simulink model "boost_converter1"  (R2022b)
settings: Solver=ode15s  StartTime=0.0  StopTime=2  RelTol=1e-3
libraries: spsSeriesRLCBranchLib x6, spsMosfetLib x5, spsCurrentMeasurementLib x4, spsVoltageMeasurementLib x4, spsPVArrayLib x1, spsDiodeLib x1, spspowerguiLib x1
settings Model: Creator=nisha  LastModifiedBy=nisha

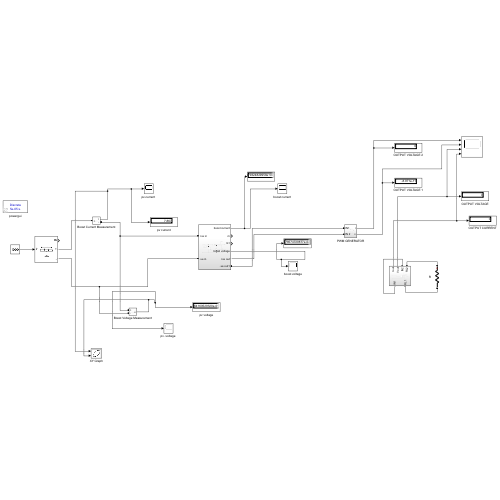
[thumbnail: Simulink's stored preview of the top-level diagram]
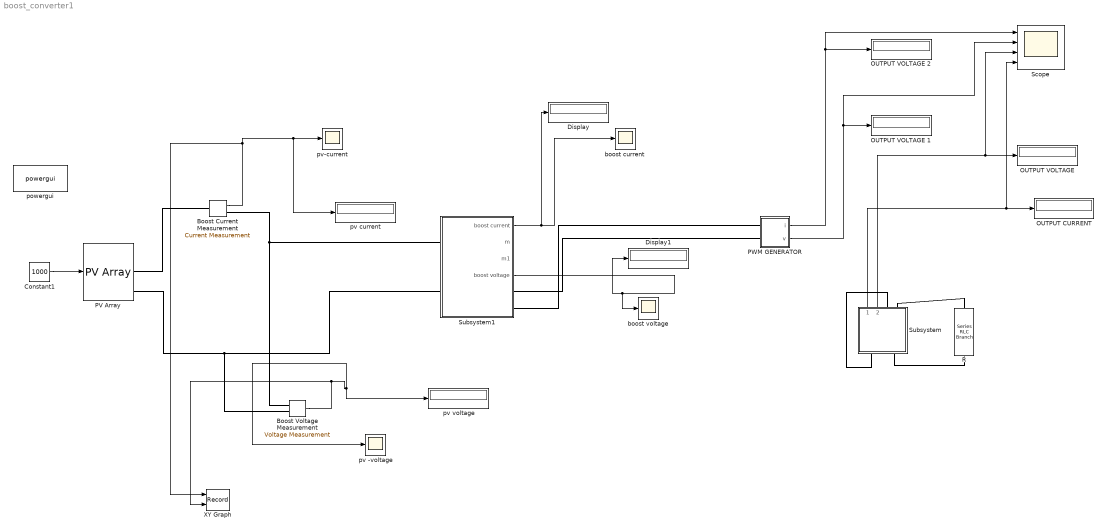
== system boost_converter1 ==
  Boost Current Measurement : spsCurrentMeasurementLib/Current Measurement  PhasorSimulation=off  OutputType=Complex  PSBequivalent=0
  Boost Voltage Measurement : spsVoltageMeasurementLib/Voltage Measurement  PhasorSimulation=off  OutputType=Complex  PSBequivalent=0
  Constant1 : Constant  Value=1000
  Display : Display
      settings: Format=long_e
  Display1 : Display
      settings: Format=long_e
  OUTPUT CURRENT : Display
  OUTPUT VOLTAGE : Display
  OUTPUT VOLTAGE 1 : Display
  OUTPUT VOLTAGE 2 : Display
  PV Array : spsPVArrayLib/PV Array  Npar=1  Nser=1  PlotType=array @ 1000 W/m2 & specified temperatures  S_vec="[ 1000  500  100 ]"  Temp_C_vec="[ 45 25  ]"  ModuleName=User-defined  PlotWhenSelected=off  Pm=213.15  Ncell=60  Voc=35  Isc=7.84  Vm=29  Im=7.35  beta_Voc_pc=-0.36099  alpha_Isc_pc=0.102  beta_Voc=-0.12635  alpha_Isc=0.0079968  IL=7.8812  I0=2.9282e-10  nI=0.94636  Rsh=184.8932  Rs=0.22133  RobustModel=on  RobustCellTemperature=25  BAL=on  Tc=1e-6  Tfilter=5e-5
  PWM GENERATOR : Subsystem
  R : spsSeriesRLCBranchLib/Series RLC Branch  LConnTagsString=__new0  RConnTagsString=__new0  BranchType=R  Resistance=1e-3  Inductance=10e-3  SetiL0=off  InitialCurrent=0  Capacitance=1e-6  Setx0=off  InitialVoltage=0  Measurements=None
  Scope : Scope  NumInputPorts=4
  Subsystem : Subsystem
  Subsystem1 : Subsystem
  XY Graph : Record  FileSettingsInternal="{\"entries\":[{\"content\":{\"excelSettings\":{\"content\":{},\"type\":\"Streamout.ExcelSettings\"}},\"type\":\"Streamout.FileSettingStorage\",\"uuid\":\"bb79825a-9a84-48d6-b614-86dd706c150b\"}],\"packageUris\":[\"http://schema.mathworks.com/mf0/streamout_blocks/R2020a\"],\"version\":\"1.0\"}"  Layout=[1 1]  SignalsInternal="{\"entries\":[{\"content\":{\"signals\":[{\"content\":{\"blockPath\":[\"boost_converter1/XY Graph\"],\"channel\":[],\"dimensions\":[1],\"domain\":\"boost_converter1/XY Graph\",\"lineColor\":\"#a2142f\",\"plots\":[1],\"port\":1,\"sid\":[],\"signalID\":8,\"signalName\":\"Boost Current Measurement\"},\"type\":\"RecordBlkView.Signal\",\"uuid\":\"aac8f88a-0a32-46b7-9f55-3afda7bd7b5f\"},{\"content\":{\"blockPath\":[\"boost_converter1/XY Graph\"],\"channel\":[],\"dimensions\":[1],\"domain\":\"boost_converter1/XY Graph\",\"lineColor\":\"#139fff\",\"plots\":[1],\"port\":2,\"sid\":[],\"signalID\":11,\"signalName\":\"Boost Voltage Measurement\"},\"type\":\"RecordBlkView.Signal\",\"uuid\":\"9a516fd9-1f24-4ca3-8a78-6277114d30cd\"}]},\"type\":\"RecordBlkView.InputSignals\",\"uuid\":\"dc6686e9-87f2-4b25-8e6b-96e90d879104\"}],\"packageUris\":[\"http://schema.mathworks.com/mf0/streamout_blocks/R2020a\"],\"version\":\"1.0\"}"  VisualizationBindings="{\"xyplotplugin\":{\"info\":[{\"series\":[{\"bindingParametersList\":[{\"parameter\":\"X-Axis\",\"signalID\":8,\"signalName\":\"Boost Current Measurement\"},{\"parameter\":\"Y-Axis\",\"signalID\":11,\"signalName\":\"Boost Voltage Measurement\"}],\"seriesID\":18183}],\"subplotID\":1}]}}"  CompatibilityTag=XY
  boost current : Scope
  boost voltage : Scope
  powergui : spspowerguiLib/powergui  Priority=1  SimulationMode=Discrete  SampleTime=5e-5  frequency=60  Iterations=50  frequencyindice=0  Pbase=100e6  ErrMax=1e-4  UnitsV=kV  UnitsW=MW  buscounter=0  FunctionMessages=off  echomessages=off  EnableUseOfTLC=off  CurrentSourceSwitches=off  DisableSnubberDevices=off  DisableRonSwitches=off  DisableVfSwitches=off  DisplayEquations=off  AutomaticDiscreteSolvers=off  SolverType=Tustin/Backward Euler (TBE)  Interpol=off  ExternalGateDelay=off  methode=off  Ts=100  x0status=blocks  SPID=on  SwTol=0  HookPort=off  NonlinearTolerance=1e-4  nMaxIteration=100  ContinueOnMaxIteration=off  RestoreLinks=warning  ResistiveCurrentMeasurement=off  Frange=[0:2:500]  Ylog=off  Xlog=on  ShowGrid=off  save=off  variable=ZData  structure=0  ZoomFFT=off  StartTime=0.0  cycles=1  DisplayStyle=1  fundamental=60  FreqAxis=off  MaxFrequency=1000  frequencyindicesteady=1  RmsSteady=1  display=off
  "pv -voltage " : Scope
  pv current : Display
  pv voltage : Display
      settings: Format=long_e
  "pv-current " : Scope
  wires:
  PWM GENERATOR/2(v) -> Scope/2, OUTPUT VOLTAGE 1/1
  PWM GENERATOR/1(i) -> Scope/1, OUTPUT VOLTAGE 2/1
  Subsystem/1(Iout) -> Scope/4, OUTPUT CURRENT/1
  Subsystem/2(Vout) -> Scope/3, OUTPUT VOLTAGE/1
  Boost Current Measurement/1 -> pv current/1, "pv-current "/1, XY Graph/1
  Constant1/1 -> PV Array/1
  Boost Voltage Measurement/1 -> XY Graph/2, "pv -voltage "/1, pv voltage/1
  Subsystem1/4(boost voltage) -> boost voltage/1, Display1/1
  Subsystem1/1(boost current) -> Display/1, boost current/1
  connections:
  R/LConn1 -- Subsystem/RConn2
  Subsystem/LConn2 -- R/RConn1
  Subsystem/LConn1 -- Subsystem/RConn1
  Boost Voltage Measurement/LConn2 -- Subsystem1/LConn2 -- PV Array/RConn2
  Boost Voltage Measurement/LConn1 -- Subsystem1/LConn1 -- Boost Current Measurement/RConn1
  PV Array/RConn1 -- Boost Current Measurement/LConn1
  Subsystem1/RConn1 -- PWM GENERATOR/LConn2
  Subsystem1/RConn2 -- PWM GENERATOR/LConn1

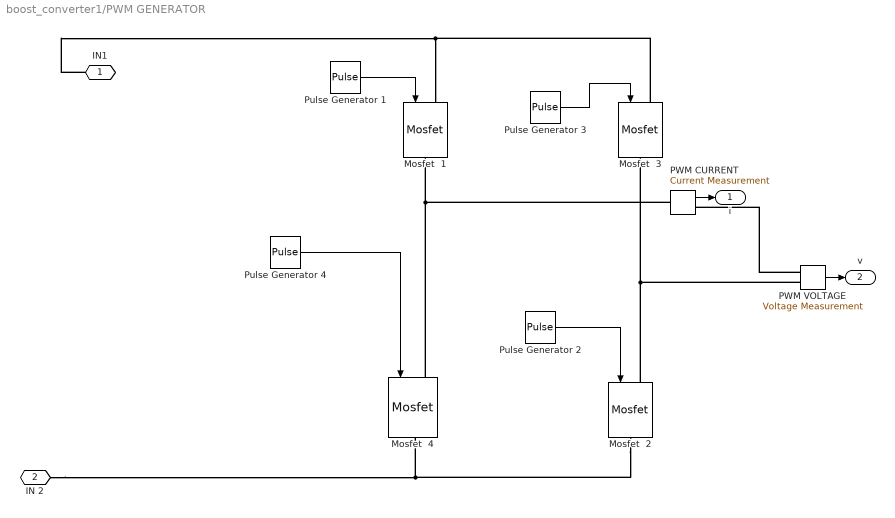
== system boost_converter1/PWM GENERATOR ==
  Mosfet  {1..4} (4 alike) : spsMosfetLib/Mosfet  Ron=0.1  Lon=0  Rd=0.01  Vfd=0  IC=0  Rs=1e5  Cs=inf  Measurements=off
  PWM CURRENT : spsCurrentMeasurementLib/Current Measurement  PhasorSimulation=off  OutputType=Complex  PSBequivalent=0
  PWM VOLTAGE : spsVoltageMeasurementLib/Voltage Measurement  PhasorSimulation=off  OutputType=Complex  PSBequivalent=0
  Pulse Generator {1..4} (4 alike) : DiscretePulseGenerator  PulseType=Time based  Period=0.02  PulseWidth=50
  "IN1 " : PMIOPort  Side=Left
  IN 2 : PMIOPort  Port=2  Side=Left
  i : Outport
  v : Outport  Port=2
  wires:
  PWM CURRENT/1 -> i/1
  Pulse Generator 3/1 -> Mosfet  3/1
  Pulse Generator 2/1 -> Mosfet  2/1
  Pulse Generator 1/1 -> Mosfet  1/1
  Pulse Generator 4/1 -> Mosfet  4/1
  PWM VOLTAGE/1 -> v/1
  connections:
  Mosfet  2/RConn1 -- Mosfet  4/RConn1 -- IN 2/RConn1
  Mosfet  3/LConn1 -- Mosfet  1/LConn1 -- "IN1 "/RConn1
  Mosfet  2/LConn1 -- Mosfet  3/RConn1 -- PWM VOLTAGE/LConn2
  Mosfet  4/LConn1 -- PWM CURRENT/LConn1 -- Mosfet  1/RConn1
  PWM VOLTAGE/LConn1 -- PWM CURRENT/RConn1

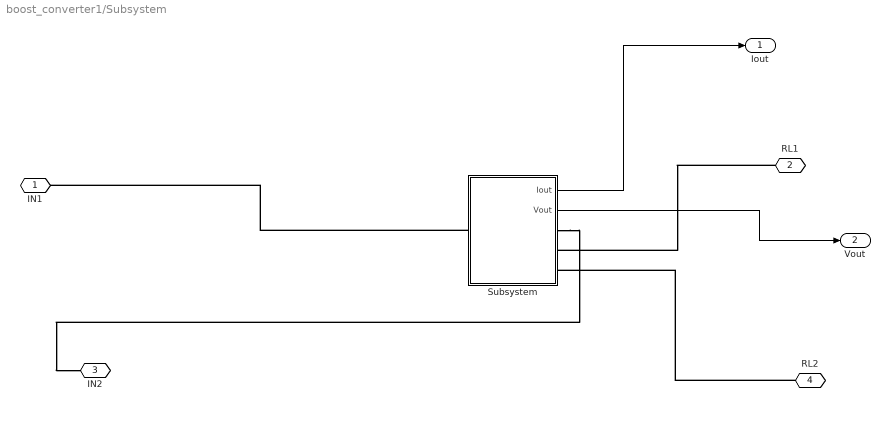
== system boost_converter1/Subsystem ==
  Subsystem : Subsystem
  "IN1 " : PMIOPort  Side=Left
  RL1 : PMIOPort  Port=2  Side=Left
  IN2 : PMIOPort  Port=3  Side=Right
  RL2 : PMIOPort  Port=4  Side=Right
  Iout : Outport
  Vout : Outport  Port=2
  wires:
  Subsystem/1(Iout) -> Iout/1
  Subsystem/2(Vout) -> Vout/1
  connections:
  Subsystem/LConn1 -- "IN1 "/RConn1
  Subsystem/RConn1 -- IN2/RConn1
  RL1/RConn1 -- Subsystem/RConn2
  RL2/RConn1 -- Subsystem/RConn3

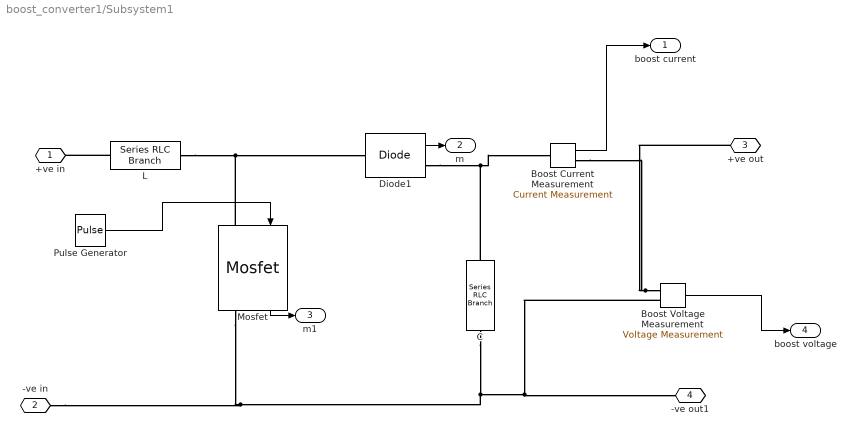
== system boost_converter1/Subsystem1 ==
  Boost Current Measurement : spsCurrentMeasurementLib/Current Measurement  PhasorSimulation=off  OutputType=Complex  PSBequivalent=0
  Boost Voltage Measurement : spsVoltageMeasurementLib/Voltage Measurement  PhasorSimulation=off  OutputType=Complex  PSBequivalent=0
  C : spsSeriesRLCBranchLib/Series RLC Branch  LConnTagsString=__new0  RConnTagsString=__new0  BranchType=C  Resistance=1e-3  Inductance=250e-6  SetiL0=off  InitialCurrent=0  Capacitance=1000e-6  Setx0=off  InitialVoltage=0  Measurements=None
  Diode1 : spsDiodeLib/Diode  Ron=0.001  Lon=0  Vf=0.8  IC=0  UseSnubber=0  Rs=500  Cs=250e-9  Measurements=on
  L : spsSeriesRLCBranchLib/Series RLC Branch  LConnTagsString=__new0  RConnTagsString=__new0  BranchType=L  Resistance=1e-3  Inductance=400e-3  SetiL0=off  InitialCurrent=0  Capacitance=1e-6  Setx0=off  InitialVoltage=0  Measurements=None
  Mosfet : spsMosfetLib/Mosfet  Ron=0.1  Lon=0  Rd=0.01  Vfd=0  IC=0  Rs=1e5  Cs=inf  Measurements=on
  Pulse Generator : DiscretePulseGenerator  PulseType=Time based  Period=10  PulseWidth=5
  +ve in : PMIOPort  Side=Left
  -ve in : PMIOPort  Port=2  Side=Left
  +ve out : PMIOPort  Port=3  Side=Right
  -ve out1 : PMIOPort  Port=4  Side=Right
  boost current : Outport
  m : Outport  Port=2
  m1 : Outport  Port=3
  boost voltage : Outport  Port=4
  wires:
  Mosfet/1 -> m1/1
  Boost Current Measurement/1 -> boost current/1
  Pulse Generator/1 -> Mosfet/1
  Boost Voltage Measurement/1 -> boost voltage/1
  Diode1/1 -> m/1
  connections:
  Mosfet/LConn1 -- L/RConn1 -- Diode1/LConn1
  Diode1/RConn1 -- C/LConn1 -- Boost Current Measurement/LConn1
  -ve in/RConn1 -- Mosfet/RConn1 -- C/RConn1 -- Boost Voltage Measurement/LConn2 -- -ve out1/RConn1
  Boost Voltage Measurement/LConn1 -- Boost Current Measurement/RConn1 -- +ve out/RConn1
  L/LConn1 -- +ve in/RConn1

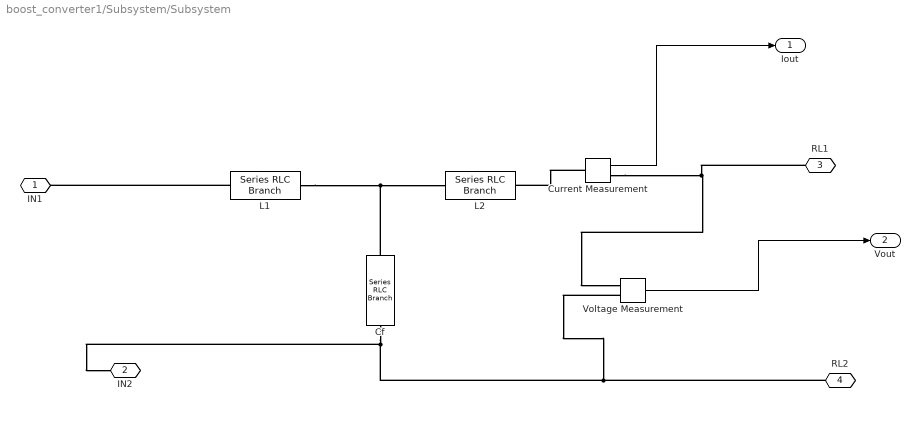
== system boost_converter1/Subsystem/Subsystem ==
  Cf : spsSeriesRLCBranchLib/Series RLC Branch  LConnTagsString=__new0  RConnTagsString=__new0  BranchType=C  Resistance=1e-3  Inductance=400e-3  SetiL0=off  InitialCurrent=0  Capacitance=680e-6  Setx0=off  InitialVoltage=0  Measurements=None
  Current Measurement : spsCurrentMeasurementLib/Current Measurement  PhasorSimulation=off  OutputType=Complex  PSBequivalent=0
  L1 : spsSeriesRLCBranchLib/Series RLC Branch  LConnTagsString=__new0  RConnTagsString=__new0  BranchType=L  Resistance=1e-3  Inductance=10e-3  SetiL0=off  InitialCurrent=0  Capacitance=1e-6  Setx0=off  InitialVoltage=0  Measurements=None
  L2 : spsSeriesRLCBranchLib/Series RLC Branch  LConnTagsString=__new0  RConnTagsString=__new0  BranchType=L  Resistance=1e-3  Inductance=10e-3  SetiL0=off  InitialCurrent=0  Capacitance=1e-6  Setx0=off  InitialVoltage=0  Measurements=None
  Voltage Measurement : spsVoltageMeasurementLib/Voltage Measurement  PhasorSimulation=off  OutputType=Complex  PSBequivalent=0
  IN1 : PMIOPort  Side=Left
  IN2 : PMIOPort  Port=2  Side=Right
  RL1 : PMIOPort  Port=3  Side=Right
  RL2 : PMIOPort  Port=4  Side=Right
  Iout : Outport
  Vout : Outport  Port=2
  wires:
  Voltage Measurement/1 -> Vout/1
  Current Measurement/1 -> Iout/1
  connections:
  Current Measurement/LConn1 -- L2/RConn1
  Current Measurement/RConn1 -- RL1/RConn1 -- Voltage Measurement/LConn1
  Cf/RConn1 -- IN2/RConn1 -- RL2/RConn1 -- Voltage Measurement/LConn2
  L1/RConn1 -- Cf/LConn1 -- L2/LConn1
  L1/LConn1 -- IN1/RConn1
